simulink model "discretething"  (R2016a)
settings: Solver=ode45  StartTime=0.0  StopTime=10.0  RelTol=1e-3
settings Model: Creator=Craig  LastModifiedBy=STEM Student
settings DataIOCC: LimitDataPoints=on  SaveFormat=Array
settings HardwareCC: ProdBitPerPointer=32  ProdLargestAtomicFloat=None  ProdIntDivRoundTo=Undefined  ProdEndianess=Unspecified  ProdWordSize=32  ProdHWDeviceType=32-bit Generic
settings ModelReferenceCC: PropagateSignalLabelsOutOfModel=off
settings ConfigComp: CovModelRefEnable=Off

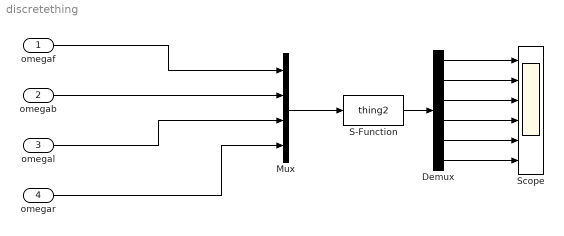
== system discretething ==
  omegaf : Inport
  omegab : Inport  Port=2
  omegal : Inport  Port=3
  omegar : Inport  Port=4
  Demux : Demux  Outputs=6
  Mux : Mux
  S-Function : S-Function  FunctionName=thing2  SFunctionDeploymentMode=off  EnableBusSupport=off
  Scope : Scope  NumInputPorts=6
  wires:
  Mux/1 -> S-Function/1
  S-Function/1 -> Demux/1
  Demux/1 -> Scope/1
  Demux/2 -> Scope/2
  Demux/3 -> Scope/3
  Demux/4 -> Scope/4
  Demux/5 -> Scope/5
  Demux/6 -> Scope/6
  omegaf/1 -> Mux/1
  omegab/1 -> Mux/2
  omegal/1 -> Mux/3
  omegar/1 -> Mux/4
